simulink model "Offline_DataImport_AND_Preprocessing_ECGandSCG3D"  (R2020b)
settings: Solver=FixedStepDiscrete  StartTime=0.0  StopTime=param_sim_time  FixedStep=1/fs  MaxStep=1/fs  RelTol=1e-3
undefined symbols (not defined in the file): fdesignblkfcn, fs, gcbh, param_tot_samples
(part 2 of 3)

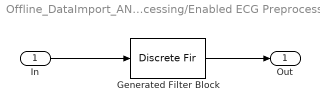
== system Offline_DataImport_AND_Preprocessing_ECGandSCG3D/ECG Preprocessing/Enabled ECG Preprocessing Subsystem/ECG Filtfiltering/Bandpass Filter 2 ==
  In : Inport
  Generated Filter Block : DiscreteFir  Tag=BlockMethodSubSystem  Coefficients=[-0.0114243088354877773 0.00587624110456374388 0.00413946068324517157 0.00264334557424035672 0.00138774422276622192 0.00039597756815762733 -0.000357391963790950132 -0.000870027328167087902 -0.00118474210009046274 -0.0013114772414377189 -0.00130211118137258525 -0.00117028348293094116 -0.000969555288066135598 -0.000709991739662891794 -0.000441672338585462343 -0.000165596169411169614 7.38618239838010476e-05 0.000289182992126718261 0.00043918297873611449 0.000554539538172022298 0.000596791094711021305 0.000591852861038305242 0.000558642096174625374 0.000449318410474004379 0.000334719809825502479 0.00020575650819831294 5.39363215079843861e-05 -0.000101322531501510382 -0.000240833690149395291 -0.000354646039305753225 -0.000451018706232981029 -0.000523127741752206499 -0.000570171746042747937 -0.000579976289078059509 -0.000560050610609794802 -0.000510203484091005868 -0.000444253999700439106 -0.000361620699264023418 -0.000270418439597897714 -0.000171285996548194847 -6.96491449474114649e-05 2.51074882581126674e-05 0.000107701466472475207 0.000177443554931332875 0.000215288445749358542 0.000245848468855064048 0.000245696970898627229 0.000229649686627229205 0.00019096241212286473 0.000142984412950488554 7.04459950623022302e-05 -8.24128026295257998e-06 -9.80593727097200246e-05 -0.000181512369773678683 -0.000268731962362029828 -0.000342263684306691809 -0.000409113387221587271 -0.000453067377901137172 -0.000486836085121275519 -0.000497275928952340546 -0.00049828288783324709 -0.000472232231767717378 -0.00043821960462679492 -0.000378588991066479766 -0.000316844305738618603 -0.000241178452312015845 -0.000166037327502541535 -8.72939132895780845e-05 -1.92312446675550752e-05 4.72061762121969014e-05 9.32922079647201252e-05 0.000128677828260322091 0.000142225646220916352 0.000145392718308013161 0.000124316294889322346 9.22525950362868691e-05 3.91139366419743922e-05 -2.09540055264127723e-05 -9.84817072707550728e-05 -0.000176447200533612 -0.000261969930569216219 -0.000338398170707415388 -0.000413673787246831778 -0.000474956484152477126 -0.000526126847064748229 -0.000557031780194342657 -0.000573463759814568652 -0.000565518328802135789 -0.000545968260267525388 -0.000503292825521842527 -0.000450686144492560767 -0.00038193732270500047 -0.000310533512604118864 -0.000229221000311531989 -0.000153634622944792687 -7.7008709436998668e-05 -1.29951882972875049e-05 4.41972427699440645e-05 7.97744827227258452e-05 0.000101355022460052069 9.88614688825825011e-05 8.13696224336354218e-05 3.98982051577762009e-05 -1.42484593806998378e-05 -8.82654671942838254e-05 -0.000167074457359766074 -0.00025963077237387 -0.000347989994374806391 -0.000439444994547399936 -0.00051811479354047299 -0.000590082617058047473 -0.000641838802120880611 -0.000681503522967578934 -0.000694804478821137508 -0.00069209853970065606 -0.000663795693677639645 -0.000621757222242421206 -0.000557224399686986893 -0.000484587241980041772 -0.000396687438130890677 -0.000308737174406251494 -0.000214743893139471981 -0.00013218336614707546 -5.38482479860227792e-05 3.99111044497961476e-06 4.92154210607297082e-05 6.74354760492514721e-05 6.74472479585495194e-05 4.02217001782036176e-05 -4.06942016077313506e-06 -7.33562872444193381e-05 -0.000154074998390272069 -0.000252782754343081062 -0.000354062465090758047 -0.000462222943123069205 -0.000562271536985421011 -0.000658661832374597689 -0.000735808311790427799 -0.000799943578584080828 -0.000838241882526128551 -0.000857844739487072239 -0.000847533102258754556 -0.000817418121589637975 -0.000760200301916437102 -0.000687422833072246636 -0.000595027809558780832 -0.000496080524377292761 -0.000387710990138089018 -0.000284208196984854847 -0.000182518571703508756 -9.84384035011120345e-05 -2.73607674165961268e-05 1.77508990696524649e-05 4.21653277528823839e-05 3.53040248291924125e-05 5.59921773045889137e-06 -5.46825757556310132e-05 -0.000133739024050423885 -0.000236066993422962002 -0.000348549704079315764 -0.000473403235651745358 -0.000595572390038458938 -0.000716976323207035166 ...(+20655 chars)]  InputProcessing=Columns as channels (frame based)
  Out : Outport  VectorParamsAs1DForOutWhenUnconnected=off
  wires:
  Generated Filter Block/1 -> Out/1
  In/1 -> Generated Filter Block/1

== system Offline_DataImport_AND_Preprocessing_ECGandSCG3D/SCG Preprocessing/Enabled SCG Preprocessing Subsystem/Filtfiltering/Bandpass Filter 1 ==
  In : Inport
  Generated Filter Block : DiscreteFir  Tag=BlockMethodSubSystem  Coefficients=[-0.0141280809748904439 0.00296128789229228515 0.00257104999710804256 0.00216178345802768047 0.00175552729414372999 0.00135185618919184472 0.000971465225508600858 0.000611761661220453987 0.000291406420521167497 4.82187739932540826e-06 -0.000231481095028417821 -0.000426883300566277893 -0.000566810793415693445 -0.000665092291782963183 -0.000708283395739488578 -0.000716103852974601593 -0.000671547633475275477 -0.000615106494933681525 -0.000488109909377643092 -0.000390234789954030728 -0.000258144491787600308 -0.000103777427082080848 3.69273719204449291e-05 0.000160217379967343004 0.000266719346682901468 0.000355855181711899407 0.00042444354991033259 0.000465107287062647284 0.000475941357662141781 0.00045436165469465474 0.000405500722307057526 0.000332653752196140906 0.000244041476717768088 0.000145867245103578971 4.31958982817989834e-05 -5.15123314384427489e-05 -0.000142923677775342456 -0.000215518203590111396 -0.000261730266501190856 -0.000295405514048500267 -0.00029258904073516806 -0.000262673662663715293 -0.000200239042161780637 -0.000119059290944066934 -1.21322536877112308e-05 0.000106963831734476281 0.00024029907401433917 0.000369441485674023434 0.000494924114257109735 0.000600074273648323539 0.000689180050721941578 0.000747556211879763649 0.000783700181000823726 0.000783037479294958205 0.000758170640681657751 0.000702221229410942768 0.00062234914182012803 0.000526336913415673471 0.000422160757970439435 0.000311595034642000654 0.000210279303290443823 0.00012116322132581063 5.51843108115603054e-05 1.14901317571792366e-05 4.63268984915096715e-07 1.97600364122418881e-05 7.52585257248264416e-05 0.000158650819102896384 0.000270390241192549133 0.000399318062573107355 0.000542643635713839848 0.000686965575031403888 0.00082909540621049771 0.000950782043587884013 0.00105531510633344837 0.0011243012388455851 0.00116225627563770577 0.00116100403898223951 0.00112659092458904618 0.00105319818945410169 0.000953344560012697739 0.000827179974613592023 0.000689621114973500843 0.000542798204792315636 0.000403935329663590928 0.000276677120819612474 0.000176948147897270508 0.000104790831399949325 7.17507496431589453e-05 7.47958920749892953e-05 0.0001189809160239471 0.000199000478147139462 0.000312036321493172272 0.000446906185270561432 0.000599958367208563298 0.000753866459386062782 0.00090376858726108622 0.00103429112272443793 0.00114049954630186627 0.00120812081357756125 0.00123691779750273109 0.00121863837734643987 0.00115823236504885609 0.00105257319614873897 0.000912433904619841529 0.000740597166721868039 0.000552884553978793408 0.000354055164106317766 0.000163199294344686802 -1.50951637483565798e-05 -0.000162513118388487796 -0.000275080946577539037 -0.000341943188723405761 -0.000363442033376501494 -0.00033415202471282282 -0.000262311282575341045 -0.000148736623332661536 -6.29165138528280099e-06 0.000158313981566005763 0.000327534481367972377 0.000492510275335960451 0.000636058676656042071 0.000750308535347654973 0.000820834153970448691 0.000843500867080383687 0.000811058974000754968 0.000725579145441419826 0.000586861203976211943 0.000405054868711680893 0.000184940546124518629 -5.5900228056928597e-05 -0.000308204861095128652 -0.000553436858002336746 -0.000780717962187617992 -0.000972296884021763008 -0.00112115970011063791 -0.00121428591472381824 -0.00125044236292902976 -0.00122449203339279784 -0.00114390543564522537 -0.00101139494448912459 -0.000841431774385854175 -0.000642541957157717614 -0.000434750691331369996 -0.000229897013949648468 -4.78783601658636093e-05 9.9539490455416782e-05 0.000197094197447343286 0.000237758271413028577 0.00021254671910410014 0.000123930849749381497 -2.84437637916960806e-05 -0.000234134053639612275 -0.000484592671067754152 -0.000762051837015052455 -0.00105285099253676732 -0.00133585896082411525 -0.00159595443115483245 -0.00181366900494322504 -0.00197783075368637359 -0.00207501327682029293 -0.00210124750065167169 -0.00205143676620881017 -0.00193252830137258941 -0.0017485276980914212 -0.00151582984003622266 ...(+13710 chars)]  InputProcessing=Columns as channels (frame based)
  Out : Outport  VectorParamsAs1DForOutWhenUnconnected=off
  wires:
  Generated Filter Block/1 -> Out/1
  In/1 -> Generated Filter Block/1
